simulink model "simu"  (R2016b)
settings: Solver=VariableStepAuto  StartTime=0.0  StopTime=5  MaxStep=0.01  RelTol=1e-4  EnableMultiTasking=on
values from neighbouring files (symbols this model uses):
  ASmax = 180    [regu.m]
  G1 = K1/(s*(1+Tm*s))    [regu.m]
  Smax = 500    [regu.m]
  TZ1 = c2d(C_pos, Tech, 'foh')    [regu.m]
  TZ2 = c2d(C_ang, Tech, 'foh')    [regu.m]
  Vmax = -Vmax    (= -10000)    [angle.m]    (also in position.m = -250; regu.m = 18)
undefined symbols (not defined in the file or in its folder): C_ang, C_pos
libraries: simulink x8
settings Model: Creator=Biscuit  LastModifiedBy=Biscuit
settings DataIOCC: LimitDataPoints=on  SaveOutput=off  SaveTime=off
settings OptimizationCC: ExpressionDepthLimit=2147483647  LifeSpan=1
settings DebuggingCC: UnderspecifiedInitializationDetection=Classic  MergeDetectMultiDrivingBlocksExec=none  FcnCallInpInsideContextMsg=warning  AllowSymbolicDim=off  StateNameClashWarn=warning  SFUnexpectedBacktrackingDiag=warning  SFNoUnconditionalDefaultTransitionDiag=warning  SFExecutionAtInitializationDiag=none
settings GRTTargetCC: TargetLangStandard=C89/C90 (ANSI)  GeneratePreprocessorConditionals=Disable all  CombineOutputUpdateFcns=off  GRTInterface=on

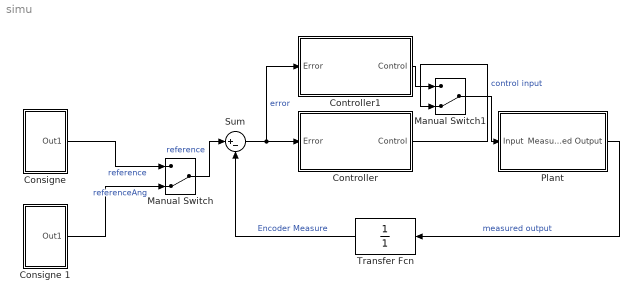
== system simu ==
  "Consigne " : Subsystem
  Consigne 1 : Subsystem
  Controller : Subsystem
  Controller1 : Subsystem
  Manual Switch : ManualSwitch  CurrentSetting=0
  Manual Switch1 : ManualSwitch  CurrentSetting=0
  Plant : Subsystem
  Sum : Sum  Inputs=|+-
  Transfer Fcn : TransferFcn  Denominator=[1]
  wires:
  Manual Switch/1 -> Sum/1  "reference"
  Plant/1(Measured Output) -> Transfer Fcn/1  "measured output"
  Sum/1 -> Controller1/1(Error), Controller/1(Error)  "error"
  Transfer Fcn/1 -> Sum/2  "Encoder Measure"
  "Consigne "/1(Out1) -> Manual Switch/1  "reference"
  Consigne 1/1(Out1) -> Manual Switch/2  "referenceAng"
  Manual Switch1/1 -> Plant/1(Input)
  Controller/1(Control) -> Manual Switch1/2  "control input"
  Controller1/1(Control) -> Manual Switch1/1

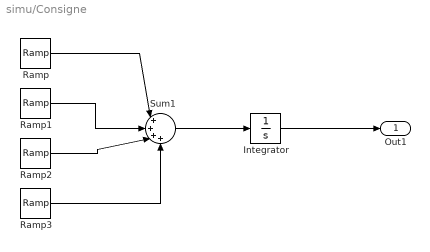
== system simu/Consigne  ==
  Integrator : Integrator
  Ramp : simulink/Sources/Ramp  slope=Smax  start=0  X0=0
  Ramp1 : simulink/Sources/Ramp  slope=-Smax  start=1  X0=0
  Ramp2 : simulink/Sources/Ramp  slope=-Smax  start=2  X0=0
  Ramp3 : simulink/Sources/Ramp  slope=Smax  start=3  X0=0
  Sum1 : Sum  Inputs=|++++
  Out1 : Outport
  wires:
  Ramp1/1 -> Sum1/2
  Ramp3/1 -> Sum1/4
  Ramp/1 -> Sum1/1
  Ramp2/1 -> Sum1/3
  Sum1/1 -> Integrator/1
  Integrator/1 -> Out1/1

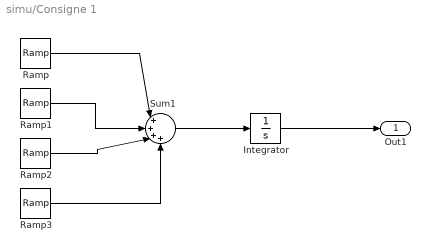
== system simu/Consigne 1 ==
  Integrator : Integrator
  Ramp : simulink/Sources/Ramp  slope=ASmax  start=0  X0=0
  Ramp1 : simulink/Sources/Ramp  slope=-ASmax  start=1  X0=0
  Ramp2 : simulink/Sources/Ramp  slope=-ASmax  start=2  X0=0
  Ramp3 : simulink/Sources/Ramp  slope=ASmax  start=3  X0=0
  Sum1 : Sum  Inputs=|++++
  Out1 : Outport
  wires:
  Ramp1/1 -> Sum1/2
  Ramp3/1 -> Sum1/4
  Ramp/1 -> Sum1/1
  Ramp2/1 -> Sum1/3
  Sum1/1 -> Integrator/1
  Integrator/1 -> Out1/1

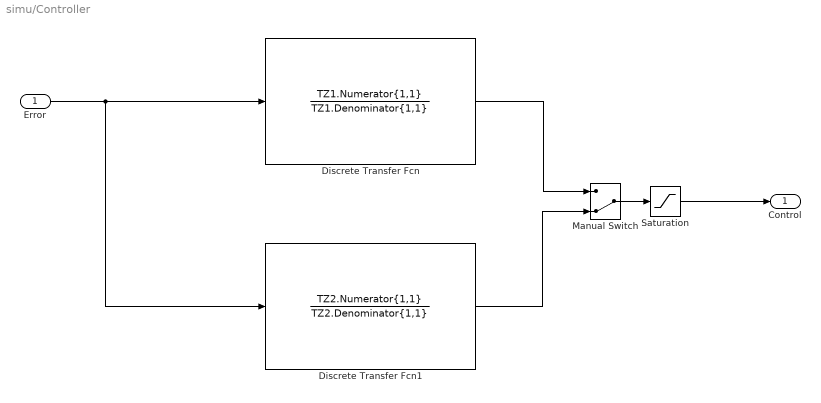
== system simu/Controller ==
  Error : Inport
  Discrete Transfer Fcn : DiscreteTransferFcn  Numerator=TZ1.Numerator{1,1}  Denominator=TZ1.Denominator{1,1}  SampleTime=TZ1.Ts
  Discrete Transfer Fcn1 : DiscreteTransferFcn  Numerator=TZ2.Numerator{1,1}  Denominator=TZ2.Denominator{1,1}  SampleTime=TZ2.Ts
  Manual Switch : ManualSwitch  CurrentSetting=0
  Saturation : Saturate  UpperLimit=Vmax  LowerLimit=-Vmax
  Control : Outport
  wires:
  Error/1 -> Discrete Transfer Fcn1/1, Discrete Transfer Fcn/1
  Discrete Transfer Fcn1/1 -> Manual Switch/2
  Discrete Transfer Fcn/1 -> Manual Switch/1
  Manual Switch/1 -> Saturation/1
  Saturation/1 -> Control/1

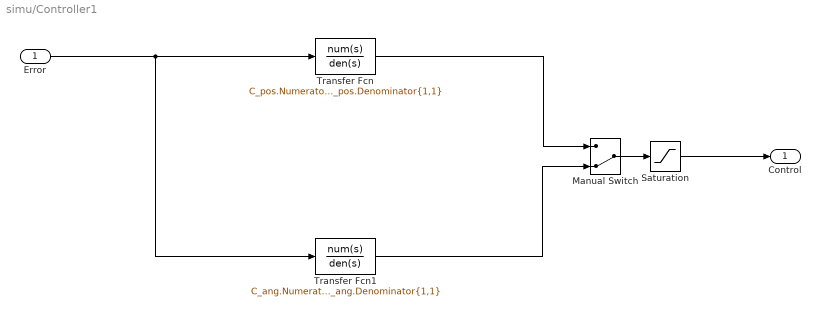
== system simu/Controller1 ==
  Error : Inport
  Manual Switch : ManualSwitch  CurrentSetting=0
  Saturation : Saturate  UpperLimit=Vmax  LowerLimit=-Vmax
  Transfer Fcn : TransferFcn  Numerator=C_pos.Numerator{1,1}  Denominator=C_pos.Denominator{1,1}
  Transfer Fcn1 : TransferFcn  Numerator=C_ang.Numerator{1,1}  Denominator=C_ang.Denominator{1,1}
  Control : Outport
  wires:
  Error/1 -> Transfer Fcn1/1, Transfer Fcn/1
  Transfer Fcn1/1 -> Manual Switch/2
  Transfer Fcn/1 -> Manual Switch/1
  Manual Switch/1 -> Saturation/1
  Saturation/1 -> Control/1

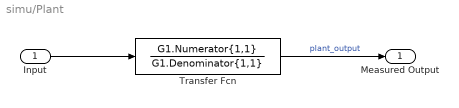
== system simu/Plant ==
  Input : Inport
  Transfer Fcn : TransferFcn  Numerator=G1.Numerator{1,1}  Denominator=G1.Denominator{1,1}
  Measured Output : Outport
  wires:
  Input/1 -> Transfer Fcn/1
  Transfer Fcn/1 -> Measured Output/1  "plant_output"
